simulink model "E2_2"  (R2022a)
settings: Solver=VariableStepAuto  StartTime=0.0  StopTime=10.0  MaxStep=.01  RelTol=1e-3
PreLoadFcn:
  | A = [-5 , 1  , 1 ;
  |       2 ,-7  , 2 ;
  |       2 , 1  ,-6 ] ;
  | B = [0   , 3.54  ;
  |      0   , 0.026 ;
  |      144 , 0.026 ] ;
  | C = [0 , 0 , 1] ;
  | D= [0] ;
  | N = obsv(A,C)
  | det (N)
  | A_ss = -6 ;
  | A_se = [1,2] ;
  | A_es = [2 ;
  |         1 ] ;
  | A_ee = [-7 , 2 ;
  |          1 ,-5 ] ;
  | B_e = [0 ,  3.54  ;
  |        0 ,  0.026 ] ;
  | B_s = [144 ,0.026 ] ;
  | C_e = [0,0] ;
  | C_s = 1 ;
  | C_re = C_s*A_se ;
  | L = [-13,13]' ;
  | A_obs = A_ee - L*C_s*A_se ;
  | B_obs= [ B_e , -L*A_ss  , A_es+L*A_ss , L*A_se ] ;
settings Model: Creator=Reza  LastModifiedBy=Reza

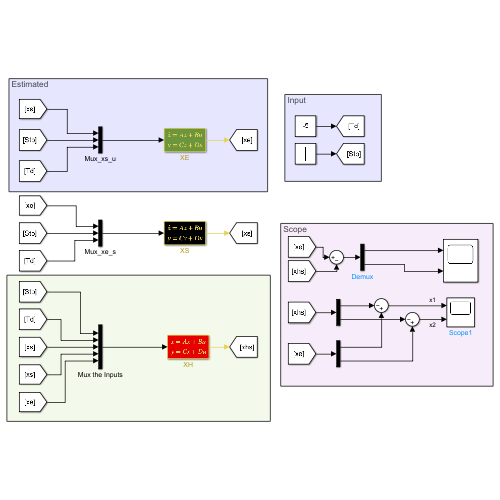
[thumbnail: Simulink's stored preview of the top-level diagram]
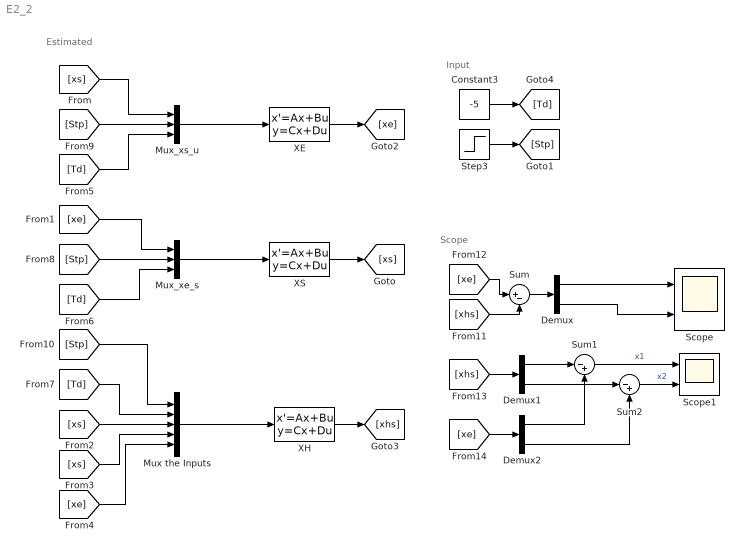
== system E2_2 ==
  note: Input
  note: Estimated
  note: Scope
  Constant3 : Constant  Value=-5
  Demux : Demux  Outputs=2
  Demux1 : Demux  Outputs=2
  Demux2 : Demux  Outputs=2
  Mux the Inputs : Mux  Inputs=5
  Mux_xe_s : Mux  Inputs=3
  Mux_xs_u : Mux  Inputs=3
  Scope : Scope  NumInputPorts=2
  Scope1 : Scope  NumInputPorts=2
  Step3 : Step  SampleTime=0
  Sum : Sum  Inputs=|+-
  Sum1 : Sum  Inputs=|-+
  Sum2 : Sum  Inputs=|-+
  XE : StateSpace  A=A_ee  B=[A_es , B_e ]  C=eye(2)  D=zeros(2,3)  InitialCondition=0  ParameterTunability=Unconstrained  AllowTunableDMatrix=on
  XH : StateSpace  A=A_obs  B=B_obs  C=eye(2,2)  D=zeros(2,6)  InitialCondition=0  ParameterTunability=Unconstrained  AllowTunableDMatrix=on
  XS : StateSpace  A=A_ss  B=[A_se , B_s]  C=eye(1)  D=zeros(1,4)  InitialCondition=0  ParameterTunability=Unconstrained  AllowTunableDMatrix=on
  wires:
  [xs] -> Mux the Inputs/4
  [Stp] -> Mux the Inputs/1
  [xs] -> Mux the Inputs/3
  [xe] -> Mux the Inputs/5
  Mux_xs_u/1 -> XE/1
  XS/1 -> [xs]
  XE/1 -> [xe]
  [xs] -> Mux_xs_u/1
  [xe] -> Mux_xe_s/1
  Mux_xe_s/1 -> XS/1
  [Stp] -> Mux_xs_u/2
  Mux the Inputs/1 -> XH/1
  [Stp] -> Mux_xe_s/2
  Constant3/1 -> [Td]
  [Td] -> Mux_xs_u/3
  [Td] -> Mux_xe_s/3
  [Td] -> Mux the Inputs/2
  XH/1 -> [xhs]
  Step3/1 -> [Stp]
  [xhs] -> Sum/2
  [xe] -> Sum/1
  Demux/1 -> Scope/1
  Sum/1 -> Demux/1
  Demux/2 -> Scope/2
  Demux1/2 -> Sum2/1
  [xhs] -> Demux1/1
  Demux1/1 -> Sum1/1
  Demux2/1 -> Sum1/2
  [xe] -> Demux2/1
  Demux2/2 -> Sum2/2
  Sum2/1 -> Scope1/2  "x2"
  Sum1/1 -> Scope1/1  "x1"
